simulink model "FlightSim"  (Simulink 7.9)
settings: Solver=ode45  StartTime=0.0  StopTime=10.0  RelTol=1e-3
undefined symbols (not defined in the file or in its folder): datcom_out, deg, ft, m, Newton, nfs, rad, Raphson, s, sigbuilder_block
libraries: aerolibconvert2 x12, aerolibadyn x2, aerolibasang x2, aerolibutil x1, simulink x1
(part 1 of 2)
settings Model: Creator=AHKh  LastModifiedBy=AHKh

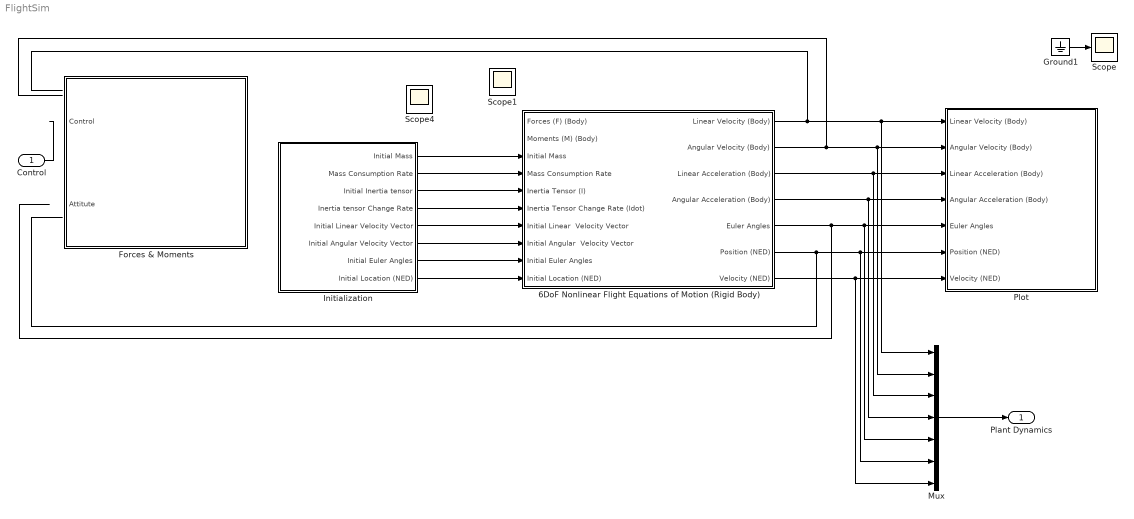
== system FlightSim ==
  Control : Inport
  6DoF Nonlinear Flight Equations of Motion (Rigid Body) : Subsystem
  Forces & Moments : Subsystem
  Ground1 : Ground
  Initialization : Subsystem
  Mux : Mux  Inputs=7
  Plot : Subsystem
  Scope : Scope
  Scope1 : Scope
  Scope4 : Scope
      settings: SaveName=ScopeData7
  Plant Dynamics : Outport
  wires:
  ? -> 6DoF Nonlinear Flight Equations of Motion (Rigid Body)/1(Forces (F) (Body)), Scope1/1
  ? -> Scope4/1, 6DoF Nonlinear Flight Equations of Motion (Rigid Body)/2(Moments (M) (Body))
  6DoF Nonlinear Flight Equations of Motion (Rigid Body)/1(Linear Velocity (Body)) -> Plot/1(Linear Velocity (Body)), Mux/1
  Initialization/3(Initial Inertia tensor) -> 6DoF Nonlinear Flight Equations of Motion (Rigid Body)/5(Inertia Tensor (I))
  Initialization/4(Inertia tensor Change Rate) -> 6DoF Nonlinear Flight Equations of Motion (Rigid Body)/6(Inertia Tensor Change Rate (Idot))
  Control/1 -> ?
  Initialization/2(Mass Consumption Rate) -> 6DoF Nonlinear Flight Equations of Motion (Rigid Body)/4(Mass Consumption Rate)
  Initialization/1(Initial Mass) -> 6DoF Nonlinear Flight Equations of Motion (Rigid Body)/3(Initial Mass)
  Initialization/5(Initial Linear Velocity Vector) -> 6DoF Nonlinear Flight Equations of Motion (Rigid Body)/7(Initial Linear  Velocity Vector)
  Initialization/6(Initial Angular Velocity Vector) -> 6DoF Nonlinear Flight Equations of Motion (Rigid Body)/8(Initial Angular  Velocity Vector)
  Initialization/7(Initial Euler Angles) -> 6DoF Nonlinear Flight Equations of Motion (Rigid Body)/9(Initial Euler Angles)
  6DoF Nonlinear Flight Equations of Motion (Rigid Body)/2(Angular Velocity (Body)) -> Plot/2(Angular Velocity (Body)), Mux/2
  6DoF Nonlinear Flight Equations of Motion (Rigid Body)/4(Angular Acceleration (Body)) -> Plot/4(Angular Acceleration (Body)), Mux/4
  Initialization/8(Initial Location (NED)) -> 6DoF Nonlinear Flight Equations of Motion (Rigid Body)/10(Initial Location (NED))
  6DoF Nonlinear Flight Equations of Motion (Rigid Body)/3(Linear Acceleration (Body)) -> Plot/3(Linear Acceleration (Body)), Mux/3
  6DoF Nonlinear Flight Equations of Motion (Rigid Body)/7(Velocity (NED)) -> Plot/7(Velocity (NED)), Mux/7
  Ground1/1 -> Scope/1
  6DoF Nonlinear Flight Equations of Motion (Rigid Body)/6(Position (NED)) -> Plot/6(Position (NED)), Mux/6
  6DoF Nonlinear Flight Equations of Motion (Rigid Body)/5(Euler Angles) -> Plot/5(Euler Angles), Mux/5
  Mux/1 -> Plant Dynamics/1

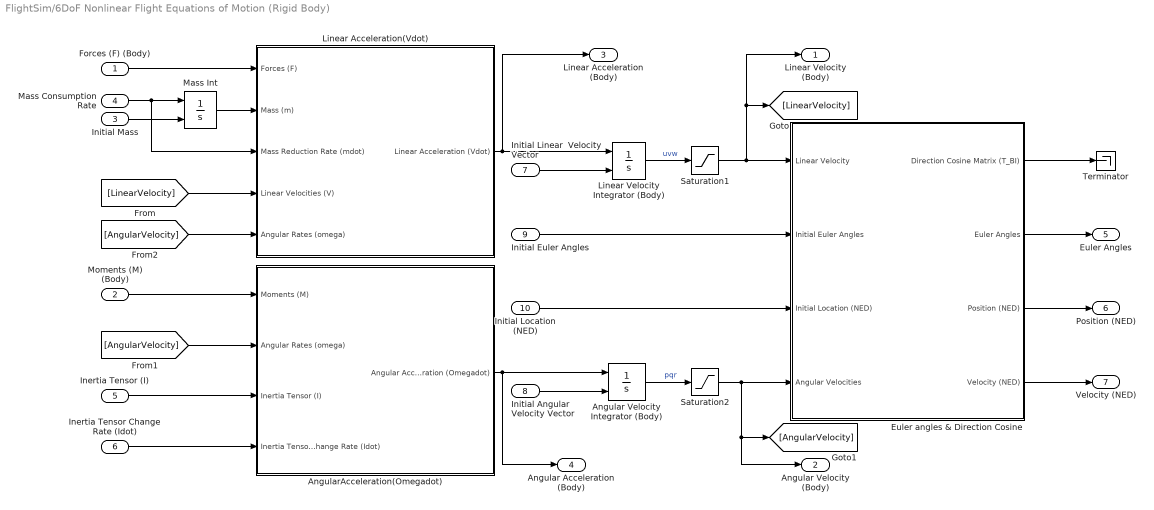
== system FlightSim/6DoF Nonlinear Flight Equations of Motion (Rigid Body) ==
  Forces (F) (Body) : Inport
  Moments (M) (Body) : Inport  Port=2  PortDimensions=[3,1]
  Initial Mass : Inport  Port=3
  Mass Consumption Rate : Inport  Port=4
  Inertia Tensor (I) : Inport  Port=5
  Inertia Tensor Change Rate (Idot) : Inport  Port=6
  Initial Linear  Velocity Vector : Inport  Port=7
  Initial Angular  Velocity Vector : Inport  Port=8
  Initial Euler Angles : Inport  Port=9
  Initial Location (NED) : Inport  Port=10
  Angular Velocity Integrator (Body) : Integrator  InitialConditionSource=external  InitialCondition=nfs.angularvel0
  AngularAcceleration(Omegadot) : Subsystem
  Euler angles & Direction Cosine : Subsystem
  Linear Acceleration(Vdot) : Subsystem
  Linear Velocity Integrator (Body) : Integrator  InitialConditionSource=external  InitialCondition=nfs.crusevelvec  ContinuousStateAttributes='BodyVelocity'
  Mass Int : Integrator  InitialConditionSource=external  InitialCondition=nfs.crusevelvec  ContinuousStateAttributes='BodyVelocity'
  Saturation1 : Saturate  UpperLimit=500  LowerLimit=-500
  Saturation2 : Saturate  UpperLimit=500  LowerLimit=-500
  Terminator : Terminator
  Linear Velocity (Body) : Outport
  Angular Velocity (Body) : Outport  Port=2
  Linear Acceleration (Body) : Outport  Port=3
  Angular Acceleration (Body) : Outport  Port=4
  Euler Angles : Outport  Port=5
  Position (NED) : Outport  Port=6
  Velocity (NED) : Outport  Port=7
  wires:
  Initial Mass/1 -> Mass Int/2
  Mass Int/1 -> Linear Acceleration(Vdot)/2(Mass (m))
  Mass Consumption Rate/1 -> Linear Acceleration(Vdot)/3(Mass Reduction Rate (mdot)), Mass Int/1
  Linear Velocity Integrator (Body)/1 -> Saturation1/1  "uvw"
  Angular Velocity Integrator (Body)/1 -> Saturation2/1  "pqr"
  Inertia Tensor (I)/1 -> AngularAcceleration(Omegadot)/3(Inertia Tensor (I))
  Inertia Tensor Change Rate (Idot)/1 -> AngularAcceleration(Omegadot)/4(Inertia Tensor Change Rate (Idot))
  Euler angles & Direction Cosine/1(Direction Cosine Matrix (T_BI)) -> Terminator/1
  Initial Location (NED)/1 -> Euler angles & Direction Cosine/3(Initial Location (NED))
  Forces (F) (Body)/1 -> Linear Acceleration(Vdot)/1(Forces (F))
  Linear Acceleration(Vdot)/1(Linear Acceleration (Vdot)) -> Linear Acceleration (Body)/1, Linear Velocity Integrator (Body)/1
  Initial Linear  Velocity Vector/1 -> Linear Velocity Integrator (Body)/2
  Initial Angular  Velocity Vector/1 -> Angular Velocity Integrator (Body)/2
  AngularAcceleration(Omegadot)/1(Angular Acceleration (Omegadot)) -> Angular Velocity Integrator (Body)/1, Angular Acceleration (Body)/1
  [LinearVelocity] -> Linear Acceleration(Vdot)/4(Linear Velocities (V))
  [AngularVelocity] -> Linear Acceleration(Vdot)/5(Angular Rates (omega))
  Moments (M) (Body)/1 -> AngularAcceleration(Omegadot)/1(Moments (M))
  [AngularVelocity] -> AngularAcceleration(Omegadot)/2(Angular Rates (omega))
  Initial Euler Angles/1 -> Euler angles & Direction Cosine/2(Initial Euler Angles)
  Euler angles & Direction Cosine/4(Velocity (NED)) -> Velocity (NED)/1
  Euler angles & Direction Cosine/2(Euler Angles) -> Euler Angles/1
  Euler angles & Direction Cosine/3(Position (NED)) -> Position (NED)/1
  Saturation1/1 -> Linear Velocity (Body)/1, [LinearVelocity], Euler angles & Direction Cosine/1(Linear Velocity)
  Saturation2/1 -> Angular Velocity (Body)/1, [AngularVelocity], Euler angles & Direction Cosine/4(Angular Velocities)

== system FlightSim/Forces & Moments ==
  Control : Inport
  Attitute : Inport  Port=2  PortDimensions=[3,1]
  Aerodynamic Forces and Moments : Subsystem  mask{datcomout=datcom_out}
      mask prompts: datcomout "DATCOM Output"
      mask Display:
      | port_label('Input',1,'V_{Body} [m/s]','texmode','on')
      | port_label('Input',2,'\omega_{Body} [rad/s]','texmode','on')
      | port_label('Input',3,'Position [m]','texmode','on')
      | port_label('Input',4,'\delta_{Control} [deg]','texmode','on')
      | port_label('Input',5,'CG [m]','texmode','on')
      | port_label('output',1,'F_{Aero} [N]','texmode','on')
      | port_label('output',2,'M_{Aero} [N.m]','texmode','on')
  Moments : Subsystem
  Repository : Subsystem
  Sum : Sum  Inputs=|++
  Thrust : Subsystem
  Weight : Subsystem
  wires:
  Weight/1(Weight) -> Sum/1
  Thrust/1(Thrust Force) -> Sum/2
  Sum/1 -> [W_T]

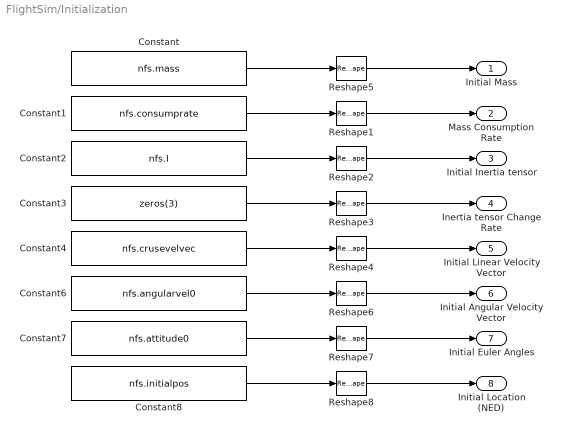
== system FlightSim/Initialization ==
  Constant : Constant  Value=nfs.mass
  Constant1 : Constant  Value=nfs.consumprate
  Constant2 : Constant  Value=nfs.I
  Constant3 : Constant  Value=zeros(3)
  Constant4 : Constant  Value=nfs.crusevelvec
  Constant6 : Constant  Value=nfs.angularvel0
  Constant7 : Constant  Value=nfs.attitude0
  Constant8 : Constant  Value=nfs.initialpos
  Reshape1 : Reshape
  Reshape2 : Reshape  OutputDimensionality=Customize  OutputDimensions=[3,3]
  Reshape3 : Reshape  OutputDimensionality=Customize  OutputDimensions=[3,3]
  Reshape{4,6..8} (4 alike) : Reshape  OutputDimensionality=Column vector (2-D)
  Reshape5 : Reshape
  Initial Mass : Outport
  Mass Consumption Rate : Outport  Port=2
  Initial Inertia tensor : Outport  Port=3
  Inertia tensor Change Rate : Outport  Port=4
  Initial Linear Velocity Vector : Outport  Port=5
  Initial Angular Velocity Vector : Outport  Port=6
  Initial Euler Angles : Outport  Port=7
  Initial Location (NED) : Outport  Port=8
  wires:
  Constant/1 -> Reshape5/1
  Constant1/1 -> Reshape1/1
  Constant2/1 -> Reshape2/1
  Constant3/1 -> Reshape3/1
  Constant4/1 -> Reshape4/1
  Constant6/1 -> Reshape6/1
  Constant7/1 -> Reshape7/1
  Constant8/1 -> Reshape8/1
  Reshape5/1 -> Initial Mass/1
  Reshape1/1 -> Mass Consumption Rate/1
  Reshape2/1 -> Initial Inertia tensor/1
  Reshape3/1 -> Inertia tensor Change Rate/1
  Reshape4/1 -> Initial Linear Velocity Vector/1
  Reshape6/1 -> Initial Angular Velocity Vector/1
  Reshape7/1 -> Initial Euler Angles/1
  Reshape8/1 -> Initial Location (NED)/1

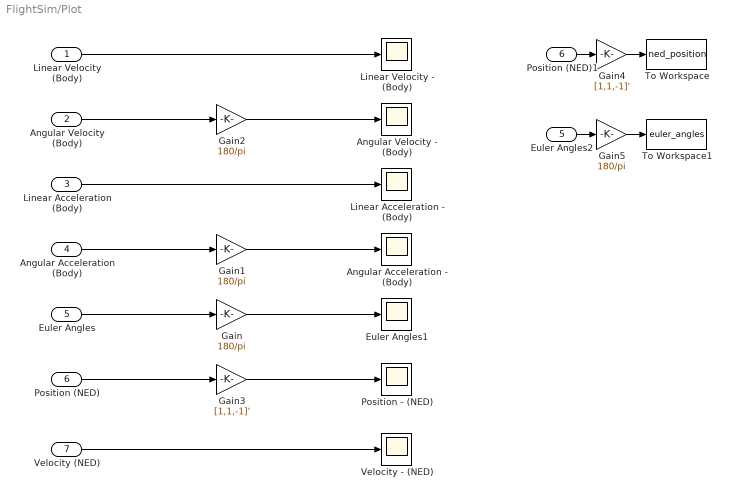
== system FlightSim/Plot ==
  Linear Velocity (Body) : Inport
  Angular Velocity (Body) : Inport  Port=2
  Linear Acceleration (Body) : Inport  Port=3
  Angular Acceleration (Body) : Inport  Port=4
  Euler Angles : Inport  Port=5  PortDimensions=3
  Position (NED) : Inport  Port=6  PortDimensions=3
  Velocity (NED) : Inport  Port=7
  Angular Acceleration - (Body) : Scope
      settings: SaveName=ScopeData17
  Angular Velocity - (Body) : Scope
      settings: SaveName=ScopeData19
  Euler Angles1 : Scope
      settings: YMin=0  YMax=2  SaveName=ScopeData3
  Euler Angles2 : InportShadow  Port=5  PortDimensions=3
  Gain{,1..2,5} (4 alike) : Gain  Gain=180/pi
  Gain3 : Gain  Gain=[1,1,-1]'
  Gain4 : Gain  Gain=[1,1,-1]'
  Linear Acceleration - (Body) : Scope
      settings: SaveName=ScopeData18
  Linear Velocity - (Body) : Scope
      settings: SaveName=ScopeData20
  Position (NED)1 : InportShadow  Port=6  PortDimensions=3
  Position - (NED) : Scope
      settings: SaveName=ScopeData2
  To Workspace : ToWorkspace  VariableName=ned_position  SampleTime=-1
  To Workspace1 : ToWorkspace  VariableName=euler_angles  SampleTime=-1
  Velocity - (NED) : Scope
      settings: SaveName=ScopeData16
  wires:
  Gain/1 -> Euler Angles1/1
  Euler Angles/1 -> Gain/1
  Position (NED)/1 -> Gain3/1
  Linear Velocity (Body)/1 -> Linear Velocity - (Body)/1
  Angular Velocity (Body)/1 -> Gain2/1
  Linear Acceleration (Body)/1 -> Linear Acceleration - (Body)/1
  Angular Acceleration (Body)/1 -> Gain1/1
  Velocity (NED)/1 -> Velocity - (NED)/1
  Gain1/1 -> Angular Acceleration - (Body)/1
  Gain2/1 -> Angular Velocity - (Body)/1
  Gain3/1 -> Position - (NED)/1
  Position (NED)1/1 -> Gain4/1
  Gain4/1 -> To Workspace/1
  Euler Angles2/1 -> Gain5/1
  Gain5/1 -> To Workspace1/1

== system FlightSim/6DoF Nonlinear Flight Equations of Motion (Rigid Body)/AngularAcceleration(Omegadot) ==
  Moments (M) : Inport  PortDimensions=[3,1]
  Angular Rates (omega) : Inport  Port=2  PortDimensions=[3,1]
  Inertia Tensor (I) : Inport  Port=3
  Inertia Tensor Change Rate (Idot) : Inport  Port=4
  Angular Rates (omega)1 : InportShadow  Port=2  PortDimensions=[3,1]
  Cross Product : Subsystem
      mask Type: Cross Product
      mask Description: Calculate the cross product of two 3-by-1 vectors.
      mask Display:
      | text(.5,.5,'Cross\nProduct\nC = AxB', ...
      | 	'HorizontalAlignment','Center',...
      | 	'VerticalAlignment','middle')
  Inertia Tensor (I)1 : InportShadow  Port=3
  Product1 : Product  Inputs=**  Multiplication=Matrix(*)  SaturateOnIntegerOverflow=on  OutDataTypeStr=Inherit: Same as first input
  Product3 : Product  Inputs=**  Multiplication=Matrix(*)  SaturateOnIntegerOverflow=on  OutDataTypeStr=Inherit: Same as first input
  Product4 : Product  Inputs=/*  Multiplication=Matrix(*)  SaturateOnIntegerOverflow=on  OutDataTypeStr=Inherit: Same as first input
  Sum1 : Sum  Inputs=|+-  SaturateOnIntegerOverflow=on
  Sum3 : Sum  Inputs=|+-  SaturateOnIntegerOverflow=on
  Angular Acceleration (Omegadot) : Outport
  wires:
  Product3/1 -> Sum1/2
  Product1/1 -> Cross Product/2(B)
  Cross Product/1(C) -> Sum3/2
  Sum1/1 -> Sum3/1
  Sum3/1 -> Product4/2
  Product4/1 -> Angular Acceleration (Omegadot)/1
  Inertia Tensor (I)1/1 -> Product4/1
  Moments (M)/1 -> Sum1/1
  Inertia Tensor Change Rate (Idot)/1 -> Product3/1
  Angular Rates (omega)/1 -> Cross Product/1(A), Product3/2
  Angular Rates (omega)1/1 -> Product1/2
  Inertia Tensor (I)/1 -> Product1/1

== system FlightSim/6DoF Nonlinear Flight Equations of Motion (Rigid Body)/Euler angles & Direction Cosine ==
  Linear Velocity : Inport  PortDimensions=[3,1]
  Initial Euler Angles : Inport  Port=2
  Initial Location (NED) : Inport  Port=3  PortDimensions=[3,1]
  Angular Velocities : Inport  Port=4
  Constant : Constant
  Euler Angles Int : Integrator  InitialConditionSource=external  InitialCondition=nfs.attitude0
  Euler angles Calculation : Subsystem
  If : If  IfExpression=u1(3)>= 0  ShowElse=off
  If Action Subsystem : Subsystem  TreatAsAtomicUnit=on
  Position Integrator : Integrator  InitialConditionSource=external  InitialCondition=[0,0,nfs.attitude0]
  Rotation Angles to DCM : Subsystem
  Selector : Selector  InputPortWidth=3  IndexOptions=Index vector (dialog)  Indices=[3 2 1]  OutputSizes=1
  Transform from Body to Inertial axes : Subsystem
      mask Display: disp('T_IB')
  Transpose : Math  Operator=transpose  SaturateOnIntegerOverflow=on
  Direction Cosine Matrix (T_BI) : Outport  PortDimensions=[3,3]
  Euler Angles : Outport  Port=2
  Position (NED) : Outport  Port=3  PortDimensions=[3,1]
  Velocity (NED) : Outport  Port=4  PortDimensions=[3,1]
  wires:
  Initial Euler Angles/1 -> Euler Angles Int/2
  Rotation Angles to DCM/1(DCM) -> Transpose/1, Direction Cosine Matrix (T_BI)/1
  Angular Velocities/1 -> Euler angles Calculation/1(Angular Velocities)
  Selector/1 -> Rotation Angles to DCM/1("[R1,R2,R3]")
  Transpose/1 -> Transform from Body to Inertial axes/1(Transformation Matrix)
  Linear Velocity/1 -> Transform from Body to Inertial axes/2(Position Vector)
  Initial Location (NED)/1 -> Position Integrator/2
  Euler Angles Int/1 -> Euler Angles/1, Selector/1, Euler angles Calculation/2(Euler Angles)
  Transform from Body to Inertial axes/1(Ve) -> Velocity (NED)/1, Position Integrator/1
  Position Integrator/1 -> Position (NED)/1, If/1
  Euler angles Calculation/1(Euler Rates) -> Euler Angles Int/1
  If/1 -> If Action Subsystem/Action
  Constant/1 -> If Action Subsystem/1(Simulation Termination)

== system FlightSim/6DoF Nonlinear Flight Equations of Motion (Rigid Body)/Linear Acceleration(Vdot) ==
  Forces (F) : Inport  PortDimensions=[3,1]
  Mass (m) : Inport  Port=2
  Mass Reduction Rate (mdot) : Inport  Port=3
  Linear Velocities (V) : Inport  Port=4  PortDimensions=[3,1]
  Angular Rates (omega) : Inport  Port=5
  Cross Product : Subsystem
      mask Type: Cross Product
      mask Description: Calculate the cross product of two 3-by-1 vectors.
      mask Display:
      | text(.5,.5,'Cross\nProduct\nC = AxB', ...
      | 	'HorizontalAlignment','Center',...
      | 	'VerticalAlignment','middle')
  Linear Velocities (V)1 : InportShadow  Port=4  PortDimensions=[3,1]
  Mass (m)1 : InportShadow  Port=2
  Product : Product  Inputs=*/  SaturateOnIntegerOverflow=on  OutDataTypeStr=Inherit: Same as first input
  Product1 : Product  Inputs=*/  SaturateOnIntegerOverflow=on  OutDataTypeStr=Inherit: Same as first input
  Product3 : Product  Inputs=**  SaturateOnIntegerOverflow=on  OutDataTypeStr=Inherit: Same as first input
  Sum1 : Sum  Inputs=|+-  SaturateOnIntegerOverflow=on
  Sum3 : Sum  Inputs=|+-  SaturateOnIntegerOverflow=on
  Linear Acceleration (Vdot) : Outport
  wires:
  Mass (m)/1 -> Product/2
  Product/1 -> Sum1/1
  Mass Reduction Rate (mdot)/1 -> Product1/1
  Mass (m)1/1 -> Product1/2
  Product1/1 -> Product3/1
  Product3/1 -> Sum1/2
  Sum1/1 -> Sum3/1
  Cross Product/1(C) -> Sum3/2
  Linear Velocities (V)/1 -> Product3/2
  Forces (F)/1 -> Product/1
  Sum3/1 -> Linear Acceleration (Vdot)/1
  Angular Rates (omega)/1 -> Cross Product/1(A)
  Linear Velocities (V)1/1 -> Cross Product/2(B)

== system FlightSim/Forces & Moments/Aerodynamic Forces and Moments ==
  Linear Velocity : Inport
  Angular Velocity : Inport  Port=2
  Position : Inport  Port=3
  Control Deflections : Inport  Port=4
  CG : Inport  Port=5
  Aero Attributes : Subsystem
  DATCOM Module : Subsystem  mask(DATCOM Module){dcase=datcomout{1}}
      mask prompts: dcase "Digital DATCOM structure"
      mask help:
      | Compute the aerodynamic forces and moments using Digital DATCOM static and dynamic stability derivatives.
      | Force Axes (Body)
      | Units (Metric)
      | Interpolation Method (Linear)
      | Extrapolation Method (Linear)
      | Out of Range Process (Linear Extrapolation)
  Demux1 : Demux  Outputs=3
  HeightInENU : Gain  Gain=-1  SaturateOnIntegerOverflow=on  OutDataTypeStr=Inherit: Same as input  ParamDataTypeStr=Inherit: Same as input
  Terminator1 : Terminator
  Terminator2 : Terminator
  Terminator3 : Terminator
  Forces (Body) : Outport
  Moments (Body) : Outport  Port=2
  wires:
  HeightInENU/1 -> Aero Attributes/2(Altitude), [Altitude]
  Demux1/2 -> Terminator3/1
  Demux1/1 -> Terminator2/1
  Demux1/3 -> HeightInENU/1
  Position/1 -> Demux1/1
  Linear Velocity/1 -> Aero Attributes/1(Linear Velocity (Body)), [LinearVelocity]
  Aero Attributes/6(Betadot) -> Terminator1/1
  Aero Attributes/1(Alpha) -> DATCOM Module/1(alp ha)
  Aero Attributes/2(Beta) -> DATCOM Module/2(beta)
  Aero Attributes/4(Dynamic Pressure) -> DATCOM Module/5(qbar)
  Aero Attributes/5(Alphadot) -> DATCOM Module/7(alpha_dot)
  Aero Attributes/3(Mach) -> DATCOM Module/3(Mach)
  Angular Velocity/1 -> DATCOM Module/8(p,q,r)
  [LinearVelocity] -> DATCOM Module/6(V)
  [Altitude] -> DATCOM Module/4(altitude)
  DATCOM Module/1(F) -> Forces (Body)/1
  DATCOM Module/2(M) -> Moments (Body)/1
  Control Deflections/1 -> DATCOM Module/9(Control Deflection)
  CG/1 -> DATCOM Module/10(CG)

== system FlightSim/Forces & Moments/Moments ==
  Linear Velocity : Inport  PortDimensions=[3,1]
  Alpha : Inport  Port=2
  Beta : Inport  Port=3
  Angular Velocity : Inport  Port=4  PortDimensions=[3,1]
  Control : Inport  Port=5
  Dynamic Pressure : Inport  Port=6
  Alphadot : Inport  Port=7
  Mach : Inport  Port=8
  "Aerodynamic Moment " : Subsystem
  Beta1 : InportShadow  Port=3
  Demux1 : Demux  Outputs=3
  Demux2 : Demux
  Linear Velocity1 : InportShadow  Port=1  PortDimensions=[3,1]
  Linear Velocity2 : InportShadow  Port=1  PortDimensions=[3,1]
  Pitch Moment Coefficient : Subsystem
  Roll Moment Coefficient : Subsystem
  Yaw Moment Coefficient : Subsystem
  Moments (Body) : Outport
  wires:
  Demux2/2 -> Pitch Moment Coefficient/5(DeltaFlap)
  Demux2/1 -> Pitch Moment Coefficient/4(DeltaElevator)
  Demux2/4 -> Yaw Moment Coefficient/6(DeltaRudder), Roll Moment Coefficient/6(DeltaRudder)
  Demux2/3 -> Yaw Moment Coefficient/5(DeltaAileron), Roll Moment Coefficient/5(DeltaAileron)
  Control/1 -> Demux2/1
  Mach/1 -> Pitch Moment Coefficient/7(Mach)
  Alphadot/1 -> Pitch Moment Coefficient/6(Alphadot)
  Demux1/2 -> Pitch Moment Coefficient/3(Q)
  Demux1/3 -> Yaw Moment Coefficient/4(R), Roll Moment Coefficient/4(R)
  Demux1/1 -> Yaw Moment Coefficient/3(P), Roll Moment Coefficient/3(P)
  Angular Velocity/1 -> Demux1/1
  Beta1/1 -> Yaw Moment Coefficient/2(beta)
  Beta/1 -> Roll Moment Coefficient/2(Beta)
  Alpha/1 -> Pitch Moment Coefficient/2(Alpha)
  Dynamic Pressure/1 -> "Aerodynamic Moment "/4(Dynamic Pressure)
  Linear Velocity2/1 -> Yaw Moment Coefficient/1(Linear Velocity)
  Linear Velocity1/1 -> Pitch Moment Coefficient/1(Linear Velocity)
  Linear Velocity/1 -> Roll Moment Coefficient/1(Linear Velocity)
  "Aerodynamic Moment "/1(Aerodynamic Moment) -> Moments (Body)/1
  Yaw Moment Coefficient/1(Cn) -> "Aerodynamic Moment "/3(Cn)
  Pitch Moment Coefficient/1(Cm) -> "Aerodynamic Moment "/2(Cm)
  Roll Moment Coefficient/1(Cl) -> "Aerodynamic Moment "/1(Cl)

== system FlightSim/Forces & Moments/Repository ==
  Control Forces : Subsystem  mask{wingarea=nfs.refarea, cLdelta_e=nfs.aero.cLdelta_e, cLdelta_f=nfs.aero.cLdelta_f, cDdelta_e=nfs.aero.cDdelta_e, cDdelta_f=nfs.aero.cDdelta_f, cDdelta_a=nfs.aero.cDdelta_a, cDdelta_r=nfs.aero.cDdelta_r, cYdelta_a=nfs.aero.cYdelta_a, cYdelta_r=nfs.aero.cYdelta_r}
      mask prompts: wingarea "Wing Area"; cLdelta_e "Derivation of CL w.r.t. Delta Elevator"; cLdelta_f "Derivation of CL w.r.t. Delta Flap"; cDdelta_e "Derivation of CD w.r.t. Delta Elevator"; cDdelta_f "Derivation of CD w.r.t. Delta Flap"; cDdelta_a "Derivation of CD w.r.t. Delta Aileron"; cDdelta_r "Derivation of CD w.r.t. Delta Rudder"; cYdelta_a "Derivation of CY w.r.t. Delta Aileron"; cYdelta_r "Derivation of CY w.r.t. Delta Rudder"
  Control Moments : Subsystem  mask{wingspan=nfs.span, wingarea=nfs.refarea, meanaerochord=nfs.meanchord, cldelta_a=nfs.aero.cldelta_a, cldelta_r=nfs.aero.cldelta_r, cmdelta_e=nfs.aero.cmdelta_e, cmdelta_f=nfs.aero.cmdelta_f, cndelta_a=nfs.aero.cndelta_a, cndelta_r=nfs.aero.cndelta_r}
      mask prompts: wingspan "Wing Span"; wingarea "Wing Area"; meanaerochord "Mean Aerodynamic Chord"; cldelta_a "Derivation of Cl w.r.t. Delta Aileron"; cldelta_r "Derivation of Cl w.r.t. Delta Rudder"; cmdelta_e "Derivation of Cm w.r.t. Delta Elevator"; cmdelta_f "Derivation of Cm w.r.t. Delta Flap"; cndelta_a "Derivation of Cn w.r.t. Delta Aileron"; cndelta_r "Derivation of Cn w.r.t. Delta Rudder"
  Forces : Subsystem

== system FlightSim/Forces & Moments/Thrust ==
  Manual Switch : simulink/Signal Routing/Manual Switch  sw=0  action=0  varsize=off
  Mux1 : Mux  Inputs=3
  Product : Product  RndMeth=Zero
  Signal Builder : Subsystem  Tag=STV Subsys  LoadFcn=sigbuilder_block('load');  StartFcn=sigbuilder_block('start');  StopFcn=sigbuilder_block('stop');  ClipboardFcn=sigbuilder_block('clipboard');  mask(Sigbuilder block){}
      mask help: Simulink:masks:SigbuilderBlock_MD
      mask init:
      | if ~strcmp(get_param(bdroot(gcbh),'SimulationStatus'),'stopped') tuvar = sigbuilder_block('maskInit'); end
      settings: CopyFcn=sigbuilder_block('copy');  DeleteFcn=sigbuilder_block('delete');  ModelCloseFcn=sigbuilder_block('modelClose');  PreSaveFcn=sigbuilder_block('preSave');  PauseFcn=sigbuilder_block('pause');  ContinueFcn=sigbuilder_block('continue');  NameChangeFcn=sigbuilder_block('namechange');  OpenFcn=sigbuilder_block('open',[437.25 199.5 550.5 399.75 ]);  CloseFcn=sigbuilder_block('close');
      mask Display: plot(0, 0, 100, 100,[2, 2, 32, 32, 2], [68, 8, 8, 68, 68],[32, 2], [38, 38], [32, 19, 2],[53, 60, 44], [32, 17, 17, 2],[16, 16, 31, 31]);txt = getActiveGroup(gcbh);text(2, 100, txt,'verticalAlignment', 'top');
  Throttle : Gain
  Trim Thrust1 : Constant  Value=nfs.trim.thrust*cos(nfs.tmisalign)
  Trim Thrust2 : Constant  Value=nfs.trim.thrust*sin(nfs.tmisalign)
  Trim Thrust3 : Constant  Value=0
  Trim Thrust4 : Constant
  Trim Thrust5 : Constant  Value=[0 0 0]'
  Thrust Force : Outport  PortDimensions=[3,1]
  Thrust Moment : Outport  Port=2  PortDimensions=[3,1]
  wires:
  Mux1/1 -> Throttle/1
  Trim Thrust3/1 -> Mux1/3
  Trim Thrust2/1 -> Mux1/2
  Trim Thrust1/1 -> Mux1/1
  Throttle/1 -> Product/1
  Product/1 -> Thrust Force/1
  Manual Switch/1 -> Product/2
  Signal Builder/1(ThrustDeviation) -> Manual Switch/1
  Trim Thrust4/1 -> Manual Switch/2
  Trim Thrust5/1 -> Thrust Moment/1

== system FlightSim/Forces & Moments/Weight ==
  note: theta
  note: phi
  Attitute : Inport  PortDimensions=[3,1]
  Mass : Inport  Port=2  PortDimensions=[3,1]
  Demux : Demux  Outputs=3
  Gain1 : Gain  Gain=-1
  Mux1 : Mux  Inputs=3
  Product{2..6} (5 alike) : Product  RndMeth=Zero
  Terminator4 : Terminator
  Trigonometric Function1 : Trigonometry  Operator=cos
  Trigonometric Function2 : Trigonometry
  Trigonometric Function3 : Trigonometry  Operator=cos
  Trigonometric Function4 : Trigonometry
  gravity : Gain  Gain=9.806
  Weight : Outport  PortDimensions=[3,1]
  wires:
  Mux1/1 -> Weight/1
  Product6/1 -> Mux1/3
  Product3/1 -> Mux1/2
  Product2/1 -> Mux1/1
  Trigonometric Function1/1 -> Product5/2
  Trigonometric Function4/1 -> Product4/1
  Trigonometric Function3/1 -> Product5/1, Product4/2
  Trigonometric Function2/1 -> Gain1/1
  Gain1/1 -> Product2/1
  Demux/3 -> Terminator4/1
  Attitute/1 -> Demux/1
  Demux/2 -> Trigonometric Function3/1, Trigonometric Function2/1
  Demux/1 -> Trigonometric Function1/1, Trigonometric Function4/1
  Mass/1 -> gravity/1
  gravity/1 -> Product6/1, Product2/2, Product3/2
  Product5/1 -> Product6/2
  Product4/1 -> Product3/1

== system FlightSim/6DoF Nonlinear Flight Equations of Motion (Rigid Body)/AngularAcceleration(Omegadot)/Cross Product ==
  A : Inport
  B : Inport  Port=2
  "A " : InportShadow  Port=1
  "B " : InportShadow  Port=2
  Subsystem2 : Subsystem
  Subsystem3 : Subsystem
  Sum : Sum  Inputs=+|-  SaturateOnIntegerOverflow=on  InputSameDT=on  OutDataTypeStr=Inherit: Same as first input
  C : Outport
  wires:
  Subsystem3/1(Out2) -> Sum/2
  Subsystem2/1(Out1) -> Sum/1
  A/1 -> Subsystem2/1(A)
  B/1 -> Subsystem2/2(B)
  Sum/1 -> C/1
  "A "/1 -> Subsystem3/1(A)
  "B "/1 -> Subsystem3/2(B)

== system FlightSim/6DoF Nonlinear Flight Equations of Motion (Rigid Body)/Euler angles & Direction Cosine/Euler angles Calculation ==
  Angular Velocities : Inport  PortDimensions=[3,1]
  Euler Angles : Inport  Port=2
  Mux1 : Mux  Inputs=[3 3 3]
  Mux2 : Mux  Inputs=3
  phidot : Fcn  Expr=u[1]+(u[2]*u[4]+u[3]*u[7])*(u[5]/u[8])
  psidot : Fcn  Expr=(u[2]*u[4]+u[3]*u[7])/u[8]
  sincos : Trigonometry  Operator=sincos
  thetadot : Fcn  Expr=u[2]*u[7]-u[3]*u[4]
  Euler Rates : Outport  PortDimensions=[3,1]  InitialOutput=0
  wires:
  sincos/2 -> Mux1/3
  sincos/1 -> Mux1/2
  Mux2/1 -> Euler Rates/1
  phidot/1 -> Mux2/1
  thetadot/1 -> Mux2/2
  psidot/1 -> Mux2/3
  Euler Angles/1 -> sincos/1
  Angular Velocities/1 -> Mux1/1
  Mux1/1 -> psidot/1, phidot/1, thetadot/1

== system FlightSim/6DoF Nonlinear Flight Equations of Motion (Rigid Body)/Euler angles & Direction Cosine/If Action Subsystem ==
  Simulation Termination : Inport
  Action Port : ActionPort  ActionType=then
  Stop Simulation : Stop
  wires:
  Simulation Termination/1 -> Stop Simulation/1

== system FlightSim/6DoF Nonlinear Flight Equations of Motion (Rigid Body)/Euler angles & Direction Cosine/Rotation Angles to DCM ==
  "[R1,R2,R3]" : Inport  PortDimensions=3
  Create 3x3 Matrix : aerolibutil/Create 3x3 Matrix
  Fcn11 : Fcn  Expr=u(5)*u(4)
  Fcn12 : Fcn  Expr=u(5)*u(1)
  Fcn13 : Fcn  Expr=-u(2)
  Fcn21 : Fcn  Expr=u(3)*u(2)*u(4) - u(6)*u(1)
  Fcn22 : Fcn  Expr=u(3)*u(2)*u(1) + u(6)*u(4)
  Fcn23 : Fcn  Expr=u(3)*u(5)
  Fcn31 : Fcn  Expr=u(6)*u(2)*u(4) + u(3)*u(1)
  Fcn32 : Fcn  Expr=u(6)*u(2)*u(1) - u(3)*u(4)
  Fcn33 : Fcn  Expr=u(6)*u(5)
  Mux : Mux  Inputs=2
  sincos1 : Trigonometry  Operator=sincos
  DCM : Outport  PortDimensions=[3,3]
  wires:
  "[R1,R2,R3]"/1 -> sincos1/1
  Create 3x3 Matrix/1 -> DCM/1
  sincos1/1 -> Mux/1
  sincos1/2 -> Mux/2
  Mux/1 -> Fcn32/1, Fcn33/1, Fcn31/1, Fcn23/1, Fcn22/1, Fcn11/1, Fcn12/1, Fcn13/1, Fcn21/1
  Fcn11/1 -> Create 3x3 Matrix/1
  Fcn12/1 -> Create 3x3 Matrix/2
  Fcn13/1 -> Create 3x3 Matrix/3
  Fcn21/1 -> Create 3x3 Matrix/4
  Fcn31/1 -> Create 3x3 Matrix/7
  Fcn22/1 -> Create 3x3 Matrix/5
  Fcn23/1 -> Create 3x3 Matrix/6
  Fcn32/1 -> Create 3x3 Matrix/8
  Fcn33/1 -> Create 3x3 Matrix/9

== system FlightSim/6DoF Nonlinear Flight Equations of Motion (Rigid Body)/Euler angles & Direction Cosine/Transform from Body to Inertial axes ==
  Transformation Matrix : Inport
  Position Vector : Inport  Port=2
  Product : Product  Multiplication=Matrix(*)  SaturateOnIntegerOverflow=on  InputSameDT=on  OutDataTypeStr=Inherit: Same as first input
  Reshape1 : Reshape  OutputDimensionality=Column vector (2-D)
  Reshape2 : Reshape
  Ve : Outport
  wires:
  Reshape2/1 -> Ve/1
  Reshape1/1 -> Product/2
  Position Vector/1 -> Reshape1/1
  Transformation Matrix/1 -> Product/1
  Product/1 -> Reshape2/1

== system FlightSim/6DoF Nonlinear Flight Equations of Motion (Rigid Body)/Linear Acceleration(Vdot)/Cross Product ==
  A : Inport
  B : Inport  Port=2
  "A " : InportShadow  Port=1
  "B " : InportShadow  Port=2
  Subsystem2 : Subsystem
  Subsystem3 : Subsystem
  Sum : Sum  Inputs=+|-  SaturateOnIntegerOverflow=on  InputSameDT=on  OutDataTypeStr=Inherit: Same as first input
  C : Outport
  wires:
  Subsystem3/1(Out2) -> Sum/2
  Subsystem2/1(Out1) -> Sum/1
  A/1 -> Subsystem2/1(A)
  B/1 -> Subsystem2/2(B)
  Sum/1 -> C/1
  "A "/1 -> Subsystem3/1(A)
  "B "/1 -> Subsystem3/2(B)

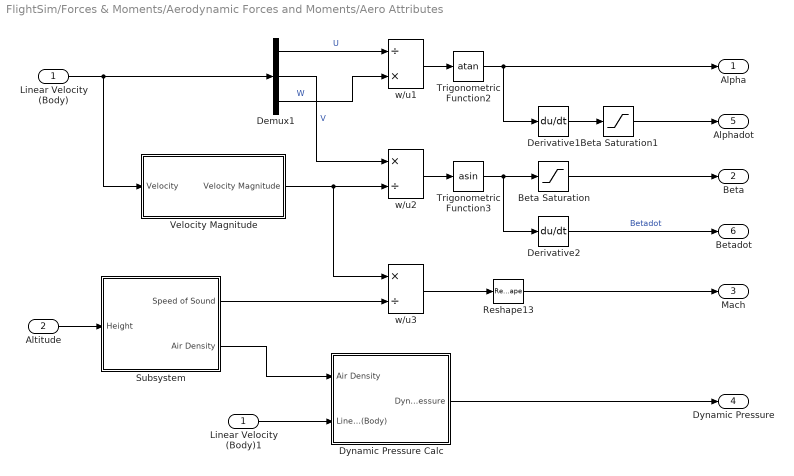
== system FlightSim/Forces & Moments/Aerodynamic Forces and Moments/Aero Attributes ==
  Linear Velocity (Body) : Inport  PortDimensions=[3,1]
  Altitude : Inport  Port=2
  Beta Saturation : Saturate  UpperLimit=5*pi/11  LowerLimit=-5*pi/11
  Beta Saturation1 : Saturate  UpperLimit=1  LowerLimit=-1
  Demux1 : Demux  Outputs=3
  Derivative1 : Derivative
  Derivative2 : Derivative
  Dynamic Pressure Calc : Subsystem
  Linear Velocity (Body)1 : InportShadow  Port=1  PortDimensions=[3,1]
  Reshape13 : Reshape
  Subsystem : Subsystem
  Trigonometric Function2 : Trigonometry  Operator=atan
  Trigonometric Function3 : Trigonometry  Operator=asin
  Velocity Magnitude : Subsystem
  w/u1 : Product  Inputs=/*  SaturateOnIntegerOverflow=on  InputSameDT=on  OutDataTypeStr=Inherit: Same as first input
  w/u2 : Product  Inputs=*/  SaturateOnIntegerOverflow=on  InputSameDT=on  OutDataTypeStr=Inherit: Same as first input
  w/u3 : Product  Inputs=*/  SaturateOnIntegerOverflow=on  InputSameDT=on  OutDataTypeStr=Inherit: Same as first input
  Alpha : Outport
  Beta : Outport  Port=2
  Mach : Outport  Port=3
  Dynamic Pressure : Outport  Port=4
  Alphadot : Outport  Port=5
  Betadot : Outport  Port=6
  wires:
  Beta Saturation1/1 -> Alphadot/1
  Subsystem/2(Air Density) -> Dynamic Pressure Calc/1(Air Density)
  Subsystem/1(Speed of Sound) -> w/u3/2
  Velocity Magnitude/1(Velocity Magnitude) -> w/u3/1, w/u2/2
  Reshape13/1 -> Mach/1
  Derivative2/1 -> Betadot/1  "Betadot"
  Beta Saturation/1 -> Beta/1
  Derivative1/1 -> Beta Saturation1/1
  Dynamic Pressure Calc/1(Dynamic Pressure) -> Dynamic Pressure/1
  Linear Velocity (Body)1/1 -> Dynamic Pressure Calc/2(Linear Velocity (Body))
  Altitude/1 -> Subsystem/1(Height)
  w/u3/1 -> Reshape13/1
  Trigonometric Function3/1 -> Beta Saturation/1, Derivative2/1
  Trigonometric Function2/1 -> Derivative1/1, Alpha/1
  w/u2/1 -> Trigonometric Function3/1
  w/u1/1 -> Trigonometric Function2/1
  Demux1/3 -> w/u1/2  "W"
  Demux1/2 -> w/u2/1  "V"
  Demux1/1 -> w/u1/1  "U"
  Linear Velocity (Body)/1 -> Velocity Magnitude/1(Velocity), Demux1/1

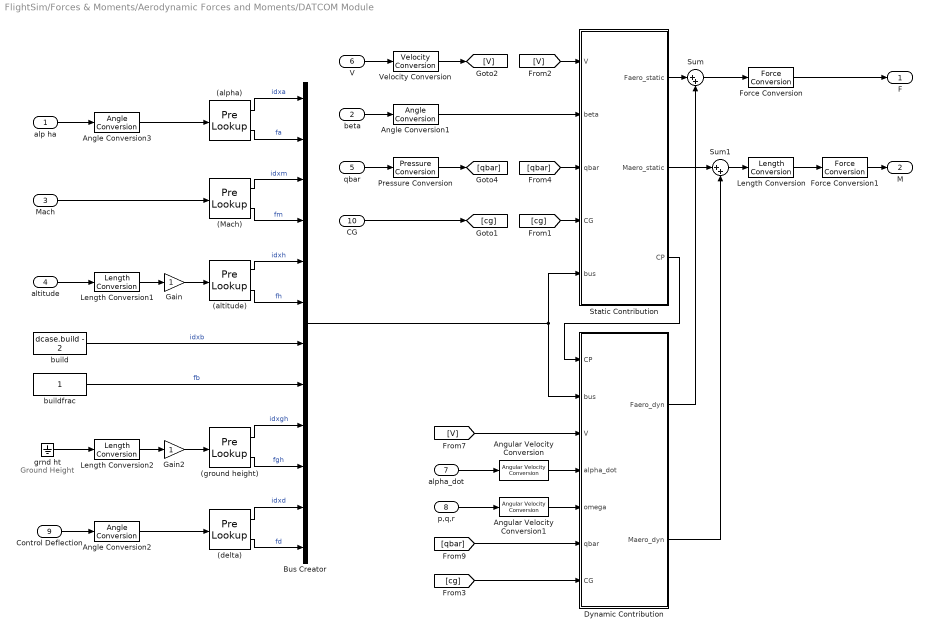
== system FlightSim/Forces & Moments/Aerodynamic Forces and Moments/DATCOM Module ==
  note: Ground
      | Height
  alp ha : Inport
  beta : Inport  Port=2
  Mach : Inport  Port=3
  altitude : Inport  Port=4
  qbar : Inport  Port=5
  V : Inport  Port=6
  alpha_dot : Inport  Port=7
  p,q,r : Inport  Port=8
  Control Deflection : Inport  Port=9
  CG : Inport  Port=10
  (Mach) : PreLookup  BreakpointsData=0:2  BeginIndexSearchUsingPreviousIndexResult=on  ExtrapMethod=Linear  IndexDataTypeStr=int32  FractionDataTypeStr=double
  (alpha) : PreLookup  BreakpointsData=dcase.alpha  BeginIndexSearchUsingPreviousIndexResult=on  ExtrapMethod=Linear  IndexDataTypeStr=int32  FractionDataTypeStr=double
  (altitude) : PreLookup  BreakpointsData=0:2  BeginIndexSearchUsingPreviousIndexResult=on  ExtrapMethod=Linear  IndexDataTypeStr=int32  FractionDataTypeStr=double
  (delta) : PreLookup  BreakpointsData=[0:2]  BeginIndexSearchUsingPreviousIndexResult=on  ExtrapMethod=Linear  IndexDataTypeStr=int32  FractionDataTypeStr=double
  (ground height) : PreLookup  BreakpointsData=[0:2]  BeginIndexSearchUsingPreviousIndexResult=on  ExtrapMethod=Linear  IndexDataTypeStr=int32  FractionDataTypeStr=double
  Angle Conversion1 : aerolibconvert2/Angle Conversion  IU=rad  OU=deg
  Angle Conversion2 : aerolibconvert2/Angle Conversion  IU=rad  OU=deg
  Angle Conversion3 : aerolibconvert2/Angle Conversion  IU=rad  OU=deg
  Angular Velocity Conversion : aerolibconvert2/Angular Velocity Conversion  IU=rad/s  OU=deg/s
  Angular Velocity Conversion1 : aerolibconvert2/Angular Velocity Conversion  IU=rad/s  OU=deg/s
  Bus Creator : BusCreator  Inputs=12
  Dynamic Contribution : Subsystem
  Force Conversion : aerolibconvert2/Force Conversion  IU=lbf  OU=N
  Force Conversion1 : aerolibconvert2/Force Conversion  IU=lbf  OU=N
  Gain : Gain
  Gain2 : Gain
  Length Conversion : aerolibconvert2/Length Conversion  IU=ft  OU=m
  Length Conversion1 : aerolibconvert2/Length Conversion  IU=m  OU=ft
  Length Conversion2 : aerolibconvert2/Length Conversion  IU=m  OU=ft
  Pressure Conversion : aerolibconvert2/Pressure Conversion  IU=Pa  OU=psf
  Static Contribution : Subsystem
  Sum : Sum  Inputs=|++
  Sum1 : Sum  Inputs=|++
  Velocity Conversion : aerolibconvert2/Velocity Conversion  IU=m/s  OU=ft/s
  build : Constant  Value=dcase.build - 2  OutDataTypeStr=int32
  buildfrac : Constant  OutDataTypeStr=double
  grnd ht : Ground
  F : Outport
  M : Outport  Port=2
  wires:
  [qbar] -> Static Contribution/3(qbar)
  Angle Conversion1/1 -> Static Contribution/2(beta)
  [V] -> Static Contribution/1("V ")
  Angle Conversion3/1 -> (alpha)/1
  (alpha)/2 -> Bus Creator/2  "fa"
  (Mach)/2 -> Bus Creator/4  "fm"
  (altitude)/2 -> Bus Creator/6  "fh"
  (altitude)/1 -> Bus Creator/5  "idxh"
  buildfrac/1 -> Bus Creator/8  "fb"
  build/1 -> Bus Creator/7  "idxb"
  (ground height)/2 -> Bus Creator/10  "fgh"
  (ground height)/1 -> Bus Creator/9  "idxgh"
  (delta)/2 -> Bus Creator/12  "fd"
  (delta)/1 -> Bus Creator/11  "idxd"
  Gain2/1 -> (ground height)/1
  Gain/1 -> (altitude)/1
  [qbar] -> Dynamic Contribution/6(qbar)
  [V] -> Dynamic Contribution/3(V)
  Velocity Conversion/1 -> [V]
  Angular Velocity Conversion1/1 -> Dynamic Contribution/5(omega)
  Angular Velocity Conversion/1 -> Dynamic Contribution/4(alpha_dot)
  Pressure Conversion/1 -> [qbar]
  Length Conversion2/1 -> Gain2/1
  Length Conversion1/1 -> Gain/1
  Length Conversion/1 -> Force Conversion1/1
  Force Conversion1/1 -> M/1
  Force Conversion/1 -> F/1
  grnd ht/1 -> Length Conversion2/1
  alpha_dot/1 -> Angular Velocity Conversion/1
  Dynamic Contribution/2(Maero_dyn) -> Sum1/2
  Static Contribution/2(Maero_static) -> Sum1/1
  Dynamic Contribution/1(Faero_dyn) -> Sum/2
  Static Contribution/1(Faero_static) -> Sum/1
  qbar/1 -> Pressure Conversion/1
  beta/1 -> Angle Conversion1/1
  Static Contribution/3("CP ") -> Dynamic Contribution/1(CP)
  p,q,r/1 -> Angular Velocity Conversion1/1
  Sum1/1 -> Length Conversion/1
  Sum/1 -> Force Conversion/1
  altitude/1 -> Length Conversion1/1
  alp ha/1 -> Angle Conversion3/1
  Mach/1 -> (Mach)/1
  (Mach)/1 -> Bus Creator/3  "idxm"
  (alpha)/1 -> Bus Creator/1  "idxa"
  Angle Conversion2/1 -> (delta)/1
  Bus Creator/1 -> Dynamic Contribution/2(bus), Static Contribution/5(bus)
  V/1 -> Velocity Conversion/1
  Control Deflection/1 -> Angle Conversion2/1
  CG/1 -> [cg]
  [cg] -> Static Contribution/4(CG)
  [cg] -> Dynamic Contribution/7(CG)

== system FlightSim/Forces & Moments/Moments/Aerodynamic Moment  ==
  Cl : Inport
  Cm : Inport  Port=2
  Cn : Inport  Port=3
  Dynamic Pressure : Inport  Port=4
  Dynamic Pressure1 : InportShadow  Port=4
  Dynamic Pressure2 : InportShadow  Port=4
  Mux : Mux  Inputs=3
  Pitch : Product  Inputs=4  SaturateOnIntegerOverflow=on  InputSameDT=on  OutDataTypeStr=Inherit: Same as first input
  Roll : Product  Inputs=4  SaturateOnIntegerOverflow=on  InputSameDT=on  OutDataTypeStr=Inherit: Same as first input
  Wing area : Constant  Value=nfs.refarea
  Wing chord : Constant  Value=nfs.meanchord
  Wing span : Constant  Value=nfs.span
  Wing span2 : Constant  Value=nfs.span
  Yaw : Product  Inputs=4  SaturateOnIntegerOverflow=on  InputSameDT=on  OutDataTypeStr=Inherit: Same as first input
  Aerodynamic Moment : Outport  PortDimensions=[3,1]
  wires:
  Yaw/1 -> Mux/3
  Pitch/1 -> Mux/2
  Roll/1 -> Mux/1
  Mux/1 -> Aerodynamic Moment/1
  Wing area/1 -> Yaw/2, Roll/2, Pitch/2
  Wing span2/1 -> Yaw/3
  Dynamic Pressure2/1 -> Yaw/1
  Dynamic Pressure1/1 -> Pitch/1
  Cl/1 -> Roll/4
  Cm/1 -> Pitch/4
  Cn/1 -> Yaw/4
  Dynamic Pressure/1 -> Roll/1
  Wing chord/1 -> Pitch/3
  Wing span/1 -> Roll/3

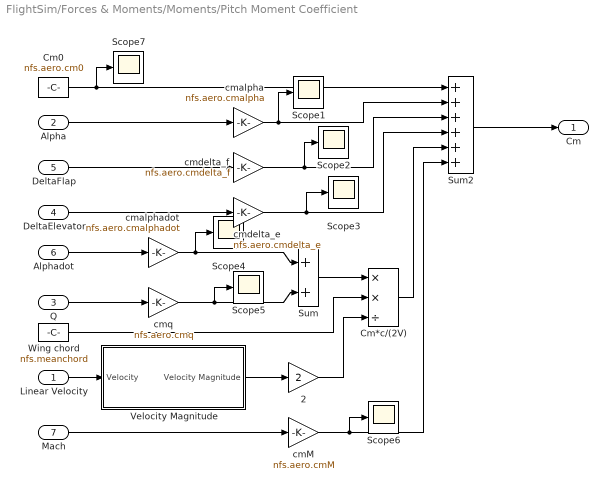
== system FlightSim/Forces & Moments/Moments/Pitch Moment Coefficient ==
  Linear Velocity : Inport
  Alpha : Inport  Port=2
  Q : Inport  Port=3
  DeltaElevator : Inport  Port=4
  DeltaFlap : Inport  Port=5
  Alphadot : Inport  Port=6  PortDimensions=1
  Mach : Inport  Port=7  PortDimensions=1
  2 : Gain  Gain=2  SaturateOnIntegerOverflow=on  OutDataTypeStr=Inherit: Same as input  ParamDataTypeStr=Inherit: Same as input
  Cm*c/(2V) : Product  Inputs=**/  SaturateOnIntegerOverflow=on  InputSameDT=on  OutDataTypeStr=Inherit: Same as first input
  Cm0 : Constant  Value=nfs.aero.cm0
  Scope{1..7} (7 alike) : Scope
      Scope1 settings: SaveName=ScopeData9
      Scope2 settings: SaveName=ScopeData11
      Scope3 settings: SaveName=ScopeData12
      Scope4 settings: SaveName=ScopeData13
      Scope5 settings: SaveName=ScopeData14
      Scope6 settings: SaveName=ScopeData15
      Scope7 settings: SaveName=ScopeData8
  Sum : Sum  SaturateOnIntegerOverflow=on  InputSameDT=on  OutDataTypeStr=Inherit: Same as first input
  Sum2 : Sum  Inputs=++++++  SaturateOnIntegerOverflow=on  InputSameDT=on  OutDataTypeStr=Inherit: Same as first input
  Velocity Magnitude : Subsystem
  Wing chord : Constant  Value=nfs.meanchord
  cmM : Gain  Gain=nfs.aero.cmM  SaturateOnIntegerOverflow=on  OutDataTypeStr=Inherit: Same as input  ParamDataTypeStr=Inherit: Same as input
  cmalpha : Gain  Gain=nfs.aero.cmalpha  SaturateOnIntegerOverflow=on  OutDataTypeStr=Inherit: Same as input  ParamDataTypeStr=Inherit: Same as input
  cmalphadot : Gain  Gain=nfs.aero.cmalphadot  SaturateOnIntegerOverflow=on  OutDataTypeStr=Inherit: Same as input  ParamDataTypeStr=Inherit: Same as input
  cmdelta_e : Gain  Gain=nfs.aero.cmdelta_e  SaturateOnIntegerOverflow=on  OutDataTypeStr=Inherit: Same as input  ParamDataTypeStr=Inherit: Same as input
  cmdelta_f : Gain  Gain=nfs.aero.cmdelta_f  SaturateOnIntegerOverflow=on  OutDataTypeStr=Inherit: Same as input  ParamDataTypeStr=Inherit: Same as input
  cmq : Gain  Gain=nfs.aero.cmq  SaturateOnIntegerOverflow=on  OutDataTypeStr=Inherit: Same as input  ParamDataTypeStr=Inherit: Same as input
  Cm : Outport  PortDimensions=1
  wires:
  Sum2/1 -> Cm/1
  Mach/1 -> cmM/1
  Q/1 -> cmq/1
  Alphadot/1 -> cmalphadot/1
  DeltaElevator/1 -> cmdelta_e/1
  DeltaFlap/1 -> cmdelta_f/1
  Alpha/1 -> cmalpha/1
  Velocity Magnitude/1(Velocity Magnitude) -> 2/1
  Linear Velocity/1 -> Velocity Magnitude/1(Velocity)
  cmM/1 -> Sum2/6, Scope6/1
  Cm*c/(2V)/1 -> Sum2/5
  cmdelta_e/1 -> Sum2/4, Scope3/1
  cmdelta_f/1 -> Sum2/3, Scope2/1
  cmalpha/1 -> Sum2/2, Scope1/1
  Cm0/1 -> Sum2/1, Scope7/1
  Sum/1 -> Cm*c/(2V)/1
  cmalphadot/1 -> Sum/1, Scope4/1
  cmq/1 -> Sum/2, Scope5/1
  Wing chord/1 -> Cm*c/(2V)/2
  2/1 -> Cm*c/(2V)/3

== system FlightSim/Forces & Moments/Moments/Roll Moment Coefficient ==
  Linear Velocity : Inport
  Beta : Inport  Port=2  PortDimensions=1
  P : Inport  Port=3
  R : Inport  Port=4
  DeltaAileron : Inport  Port=5
  DeltaRudder : Inport  Port=6
  2 : Gain  Gain=2  SaturateOnIntegerOverflow=on  OutDataTypeStr=Inherit: Same as input  ParamDataTypeStr=Inherit: Same as input
  Cl*b/(2V) : Product  Inputs=**/  SaturateOnIntegerOverflow=on  InputSameDT=on  OutDataTypeStr=Inherit: Same as first input
  Sum : Sum  SaturateOnIntegerOverflow=on  InputSameDT=on  OutDataTypeStr=Inherit: Same as first input
  Sum2 : Sum  Inputs=++++  SaturateOnIntegerOverflow=on  InputSameDT=on  OutDataTypeStr=Inherit: Same as first input
  Velocity Magnitude : Subsystem
  Wing span : Constant  Value=nfs.span
  clbeta : Gain  Gain=nfs.aero.clbeta  SaturateOnIntegerOverflow=on  OutDataTypeStr=Inherit: Same as input  ParamDataTypeStr=Inherit: Same as input
  cldelta_a : Gain  Gain=nfs.aero.cldelta_a  SaturateOnIntegerOverflow=on  OutDataTypeStr=Inherit: Same as input  ParamDataTypeStr=Inherit: Same as input
  cldelta_r : Gain  Gain=nfs.aero.cldelta_r  SaturateOnIntegerOverflow=on  OutDataTypeStr=Inherit: Same as input  ParamDataTypeStr=Inherit: Same as input
  clp : Gain  Gain=nfs.aero.clp  SaturateOnIntegerOverflow=on  OutDataTypeStr=Inherit: Same as input  ParamDataTypeStr=Inherit: Same as input
  clr : Gain  Gain=nfs.aero.clr  SaturateOnIntegerOverflow=on  OutDataTypeStr=Inherit: Same as input  ParamDataTypeStr=Inherit: Same as input
  Cl : Outport  PortDimensions=1
  wires:
  Sum2/1 -> Cl/1
  R/1 -> clr/1
  P/1 -> clp/1
  DeltaRudder/1 -> cldelta_r/1
  DeltaAileron/1 -> cldelta_a/1
  Beta/1 -> clbeta/1
  Velocity Magnitude/1(Velocity Magnitude) -> 2/1
  Linear Velocity/1 -> Velocity Magnitude/1(Velocity)
  Cl*b/(2V)/1 -> Sum2/4
  cldelta_r/1 -> Sum2/3
  cldelta_a/1 -> Sum2/2
  clbeta/1 -> Sum2/1
  2/1 -> Cl*b/(2V)/3
  Wing span/1 -> Cl*b/(2V)/2
  Sum/1 -> Cl*b/(2V)/1
  clr/1 -> Sum/2
  clp/1 -> Sum/1

== system FlightSim/Forces & Moments/Moments/Yaw Moment Coefficient ==
  Linear Velocity : Inport
  beta : Inport  Port=2  PortDimensions=1
  P : Inport  Port=3
  R : Inport  Port=4
  DeltaAileron : Inport  Port=5
  DeltaRudder : Inport  Port=6
  2 : Gain  Gain=2  SaturateOnIntegerOverflow=on  OutDataTypeStr=Inherit: Same as input  ParamDataTypeStr=Inherit: Same as input
  Cn*b/(2V) : Product  Inputs=**/  SaturateOnIntegerOverflow=on  InputSameDT=on  OutDataTypeStr=Inherit: Same as first input
  Sum : Sum  SaturateOnIntegerOverflow=on  InputSameDT=on  OutDataTypeStr=Inherit: Same as first input
  Sum2 : Sum  Inputs=++++  SaturateOnIntegerOverflow=on  InputSameDT=on  OutDataTypeStr=Inherit: Same as first input
  Velocity Magnitude : Subsystem
  Wing span : Constant  Value=nfs.span
  cnbeta : Gain  Gain=nfs.aero.cnbeta  SaturateOnIntegerOverflow=on  OutDataTypeStr=Inherit: Same as input  ParamDataTypeStr=Inherit: Same as input
  cndelta_a : Gain  Gain=nfs.aero.cndelta_a  SaturateOnIntegerOverflow=on  OutDataTypeStr=Inherit: Same as input  ParamDataTypeStr=Inherit: Same as input
  cndelta_r : Gain  Gain=nfs.aero.cndelta_r  SaturateOnIntegerOverflow=on  OutDataTypeStr=Inherit: Same as input  ParamDataTypeStr=Inherit: Same as input
  cnp : Gain  Gain=nfs.aero.cnp  SaturateOnIntegerOverflow=on  OutDataTypeStr=Inherit: Same as input  ParamDataTypeStr=Inherit: Same as input
  cnr : Gain  Gain=nfs.aero.cnr  SaturateOnIntegerOverflow=on  OutDataTypeStr=Inherit: Same as input  ParamDataTypeStr=Inherit: Same as input
  Cn : Outport  PortDimensions=1
  wires:
  Sum2/1 -> Cn/1
  R/1 -> cnr/1
  P/1 -> cnp/1
  DeltaRudder/1 -> cndelta_r/1
  DeltaAileron/1 -> cndelta_a/1
  beta/1 -> cnbeta/1
  Velocity Magnitude/1(Velocity Magnitude) -> 2/1
  Linear Velocity/1 -> Velocity Magnitude/1(Velocity)
  cnp/1 -> Sum/1
  cnr/1 -> Sum/2
  Sum/1 -> Cn*b/(2V)/1
  Wing span/1 -> Cn*b/(2V)/2
  2/1 -> Cn*b/(2V)/3
  cnbeta/1 -> Sum2/1
  cndelta_a/1 -> Sum2/2
  cndelta_r/1 -> Sum2/3
  Cn*b/(2V)/1 -> Sum2/4

== system FlightSim/Forces & Moments/Repository/Control Forces ==
  Alpha : Inport  PortDimensions=1
  Beta : Inport  Port=2
  Control : Inport  Port=3  PortDimensions=[4,1]
  Dynamic Pressure : Inport  Port=4
  Aerodynamic  Force : Subsystem  mask{wing_area=wingarea}
      mask prompts: wing_area "Wing Area"
  Demux4 : Demux
  Drag Coefficient : Subsystem  mask{cDdelta_e=cDdelta_e, cDdelta_f=cDdelta_f, cDdelta_a=cDdelta_a, cDdelta_r=cDdelta_r}
      mask prompts: cDdelta_e "Derivation of CD w.r.t. Delta Elevator"; cDdelta_f "Derivation of CD w.r.t. Delta Flap"; cDdelta_a "Derivation of CD w.r.t. Delta Aileron"; cDdelta_r "Derivation of CD w.r.t. Delta Rudder"
  Lift Coefficient : Subsystem  mask{cLdelta_e=cLdelta_e, cLdelta_f=cLdelta_f}
      mask prompts: cLdelta_e "Derivation of CL w.r.t. Delta Elevator"; cLdelta_f "Derivation of CL w.r.t. Delta Flap"
  SideForce Coefficient : Subsystem  mask{cYdelta_a=cYdelta_a, cYdelta_r=cYdelta_r}
      mask prompts: cYdelta_a "Derivation of CY w.r.t. Delta Aileron"; cYdelta_r "Derivation of CY w.r.t. Delta Rudder"
  Forces (Body) : Outport
  wires:
  Beta/1 -> Aerodynamic  Force/6(Beta)
  Alpha/1 -> Aerodynamic  Force/5(Alpha)
  Dynamic Pressure/1 -> Aerodynamic  Force/4(Dynamic Pressure)
  Demux4/4 -> SideForce Coefficient/2(DeltaRudder), Drag Coefficient/4(DeltaRudder)
  Demux4/3 -> SideForce Coefficient/1(DeltaAileron), Drag Coefficient/3(DeltaAileron)
  Demux4/2 -> Drag Coefficient/2(DeltaFlap), Lift Coefficient/2(DeltaFlap)
  Demux4/1 -> Drag Coefficient/1(DeltaElevator), Lift Coefficient/1(DeltaElevator)
  Control/1 -> Demux4/1
  SideForce Coefficient/1(CY) -> Aerodynamic  Force/3(CY)
  Drag Coefficient/1(CD) -> Aerodynamic  Force/2(CD)
  Lift Coefficient/1(CL) -> Aerodynamic  Force/1(CL)
  Aerodynamic  Force/1(Aerodynamic Force) -> Forces (Body)/1

== system FlightSim/Forces & Moments/Repository/Control Moments ==
  Control : Inport
  Dynamic Pressure : Inport  Port=2
  "Aerodynamic Moment " : Subsystem  mask{span=wingspan, refarea=wingarea, meanchord=meanaerochord}
      mask prompts: span "Wing Spapn"; refarea "Wing Area"; meanchord "Mean Aerodynamic Chord"
  Demux2 : Demux
  Pitch Moment Coefficient : Subsystem
  Roll Moment Coefficient : Subsystem
  Yaw Moment Coefficient : Subsystem
  Moments (Body) : Outport
  wires:
  Roll Moment Coefficient/1(Cl) -> "Aerodynamic Moment "/1(Cl)
  Pitch Moment Coefficient/1(Cm) -> "Aerodynamic Moment "/2(Cm)
  Yaw Moment Coefficient/1(Cn) -> "Aerodynamic Moment "/3(Cn)
  "Aerodynamic Moment "/1(Aerodynamic Moment) -> Moments (Body)/1
  Dynamic Pressure/1 -> "Aerodynamic Moment "/4(Dynamic Pressure)
  Control/1 -> Demux2/1
  Demux2/3 -> Roll Moment Coefficient/1(DeltaAileron), Yaw Moment Coefficient/1(DeltaAileron)
  Demux2/4 -> Roll Moment Coefficient/2(DeltaRudder), Yaw Moment Coefficient/2(DeltaRudder)
  Demux2/1 -> Pitch Moment Coefficient/1(DeltaElevator)
  Demux2/2 -> Pitch Moment Coefficient/2(DeltaFlap)

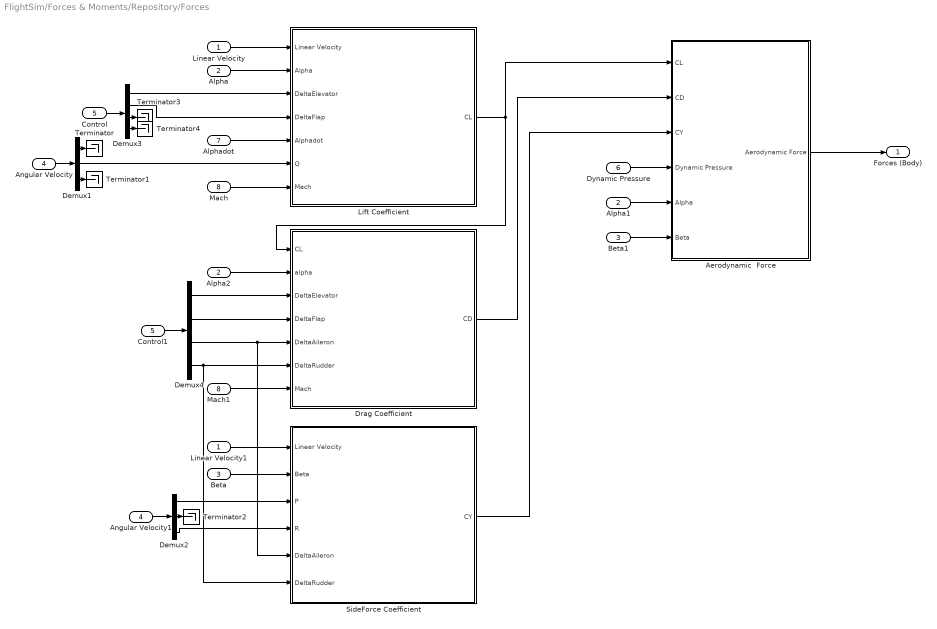
== system FlightSim/Forces & Moments/Repository/Forces ==
  Linear Velocity : Inport  PortDimensions=[3,1]
  Alpha : Inport  Port=2  PortDimensions=1
  Beta : Inport  Port=3
  Angular Velocity : Inport  Port=4  PortDimensions=[3,1]
  Control : Inport  Port=5  PortDimensions=[4,1]
  Dynamic Pressure : Inport  Port=6
  Alphadot : Inport  Port=7  PortDimensions=1
  Mach : Inport  Port=8
  Aerodynamic  Force : Subsystem
  Alpha1 : InportShadow  Port=2  PortDimensions=1
  Alpha2 : InportShadow  Port=2  PortDimensions=1
  Angular Velocity1 : InportShadow  Port=4  PortDimensions=[3,1]
  Beta1 : InportShadow  Port=3
  Control1 : InportShadow  Port=5  PortDimensions=[4,1]
  Demux1 : Demux  Outputs=3
  Demux2 : Demux  Outputs=3
  Demux3 : Demux
  Demux4 : Demux
  Drag Coefficient : Subsystem  mask{cD0=nfs.aero.cD0}
  Lift Coefficient : Subsystem  mask{cL0=nfs.aero.cL0, meanchord=nfs.meanchord}
      mask prompts: meanchord "Mean Aerodynamic Chord"
  Linear Velocity1 : InportShadow  Port=1  PortDimensions=[3,1]
  Mach1 : InportShadow  Port=8
  SideForce Coefficient : Subsystem
  Terminator{,1..4} (5 alike) : Terminator
  Forces (Body) : Outport
  wires:
  Alpha/1 -> Lift Coefficient/2(Alpha)
  Mach1/1 -> Drag Coefficient/7(Mach)
  Mach/1 -> Lift Coefficient/7(Mach)
  Alphadot/1 -> Lift Coefficient/5(Alphadot)
  Beta1/1 -> Aerodynamic  Force/6(Beta)
  Alpha1/1 -> Aerodynamic  Force/5(Alpha)
  Dynamic Pressure/1 -> Aerodynamic  Force/4(Dynamic Pressure)
  Demux4/4 -> SideForce Coefficient/6(DeltaRudder), Drag Coefficient/6(DeltaRudder)
  Demux4/3 -> SideForce Coefficient/5(DeltaAileron), Drag Coefficient/5(DeltaAileron)
  Demux4/2 -> Drag Coefficient/4(DeltaFlap)
  Demux4/1 -> Drag Coefficient/3(DeltaElevator)
  Control1/1 -> Demux4/1
  Demux3/4 -> Terminator4/1
  Demux3/3 -> Terminator3/1
  Demux3/2 -> Lift Coefficient/4(DeltaFlap)
  Demux3/1 -> Lift Coefficient/3(DeltaElevator)
  Control/1 -> Demux3/1
  Demux2/2 -> Terminator2/1
  Demux2/3 -> SideForce Coefficient/4(R)
  Demux2/1 -> SideForce Coefficient/3(P)
  Angular Velocity1/1 -> Demux2/1
  Demux1/3 -> Terminator1/1
  Demux1/1 -> Terminator/1
  Angular Velocity/1 -> Demux1/1
  Demux1/2 -> Lift Coefficient/6(Q)
  Beta/1 -> SideForce Coefficient/2(Beta)
  Linear Velocity1/1 -> SideForce Coefficient/1(Linear Velocity)
  Linear Velocity/1 -> Lift Coefficient/1(Linear Velocity)
  SideForce Coefficient/1(CY) -> Aerodynamic  Force/3(CY)
  Drag Coefficient/1(CD) -> Aerodynamic  Force/2(CD)
  Lift Coefficient/1(CL) -> Aerodynamic  Force/1(CL), Drag Coefficient/1(CL)
  Alpha2/1 -> Drag Coefficient/2(alpha)
  Aerodynamic  Force/1(Aerodynamic Force) -> Forces (Body)/1

== system FlightSim/Forces & Moments/Thrust/Signal Builder ==
  Demux : Demux  Tag=STV Demux  Outputs=1
  FromWs : FromWorkspace  Tag=STV FromWs  VariableName=tuvar  SampleTime=0  SigBuilderData=DataTag0  VnvData=DataTag1
      SigBuilderData=|
      | common.afterFinalStr = 'Extrapolate'
      | common.sampleTime = 0
      | dataSet.timeRange = [0 1200]
      | dataSet.name = 'Thrust Deviation'
      | sbobj.Groups.Name = 'Thrust Deviation'
      | sbobj.Groups.Signals.Name = 'ThrustDeviation'
      | sbobj.Groups.Signals.XData = [0 10 10 12 12 1200]
      | sbobj.Groups.Signals.YData = [1 1 1.05 1.05 1 1]
      | sbobj.Groups.TimeRange = [0 1200]
  ThrustDeviation : Outport  Tag=STV Outport
  wires:
  Demux/1 -> ThrustDeviation/1
  FromWs/1 -> Demux/1

== system FlightSim/6DoF Nonlinear Flight Equations of Motion (Rigid Body)/AngularAcceleration(Omegadot)/Cross Product/Subsystem2 ==
  A : Inport
  B : Inport  Port=2
  Demux : Demux  Outputs=3
  Demux1 : Demux  Outputs=3
  Mux : Mux  Inputs=3
  i x j : Product  SaturateOnIntegerOverflow=on  InputSameDT=on  OutDataTypeStr=Inherit: Same as first input
  j x k : Product  SaturateOnIntegerOverflow=on  InputSameDT=on  OutDataTypeStr=Inherit: Same as first input
  k x i : Product  SaturateOnIntegerOverflow=on  InputSameDT=on  OutDataTypeStr=Inherit: Same as first input
  Out1 : Outport
  wires:
  Demux1/3 -> j x k/2
  Demux/2 -> j x k/1
  Demux/3 -> k x i/1
  Demux1/1 -> k x i/2
  Demux1/2 -> i x j/2
  Demux/1 -> i x j/1
  i x j/1 -> Mux/3
  k x i/1 -> Mux/2
  j x k/1 -> Mux/1
  B/1 -> Demux1/1
  A/1 -> Demux/1
  Mux/1 -> Out1/1
